simulink model "diplomovka"  (R2014b)
settings: Solver=ode4  StartTime=0.0  StopTime=1000  FixedStep=0.5  RelTol=1e-3
libraries: fuzblock x4
settings Model: Creator=Štefan  LastModifiedBy=Dominik
settings DataIOCC: LimitDataPoints=off

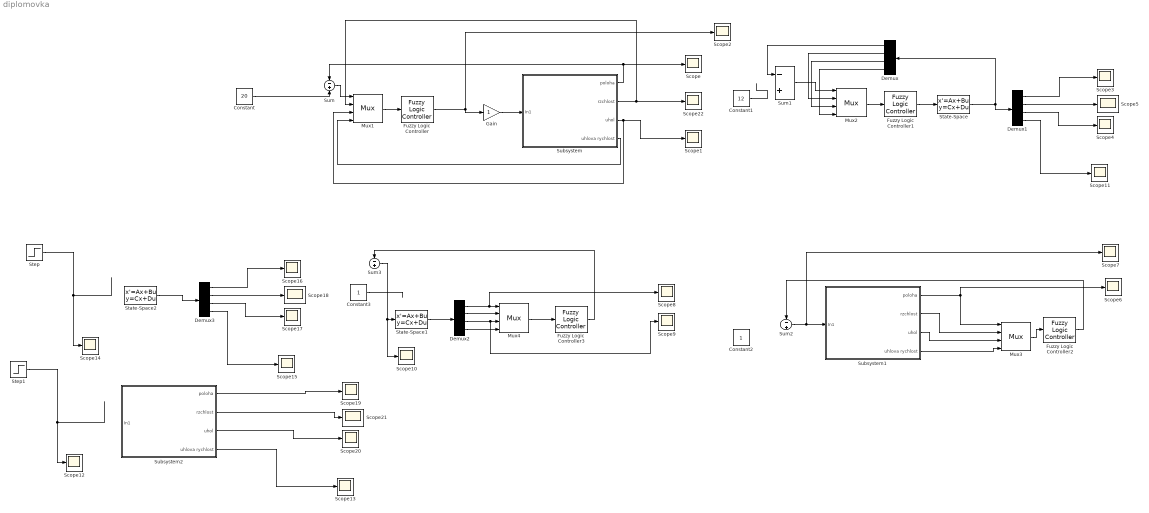
== system diplomovka ==
  Constant : Constant  Value=20
  Constant1 : Constant  Value=12
  Constant2 : Constant
  Constant3 : Constant
  Demux{,1..3} (4 alike) : Demux
  Fuzzy Logic Controller : fuzblock/Fuzzy Logic  Controller  fis=cranemajo
  Fuzzy Logic Controller1 : fuzblock/Fuzzy Logic  Controller  fis=crane
  Fuzzy Logic Controller2 : fuzblock/Fuzzy Logic  Controller  fis=crane
  Fuzzy Logic Controller3 : fuzblock/Fuzzy Logic  Controller  fis=crane
  Gain : Gain
  Mux{1..4} (4 alike) : Mux
  Scope{,1..22} (23 alike) : Scope
      Scope settings: TimeRange=1000  YMin=19.3561872909699  YMax=21.16778149386845
      Scope1 settings: YMin=-0.001  YMax=0.0004
      Scope10 settings: YMin=-0.2  YMax=1  SaveName=ScopeData10
      Scope11 settings: YMin=-0.0004  YMax=0.0004  SaveName=ScopeData11
      Scope12 settings: YMin=-0  YMax=2  SaveName=ScopeData12
      Scope13 settings: YMin=-0.0004  YMax=0.0004  SaveName=ScopeData13
      Scope14 settings: YMin=-0  YMax=2  SaveName=ScopeData14
      Scope15 settings: YMin=-0.0004  YMax=0.0004  SaveName=ScopeData15
      Scope16 settings: SaveName=ScopeData16
      Scope17 settings: SaveName=ScopeData17
      Scope18 settings: SaveName=ScopeData18
      Scope19 settings: SaveName=ScopeData19
      Scope2 settings: YMin=0  YMax=18  SaveName=ScopeData2
      Scope20 settings: SaveName=ScopeData20
      Scope21 settings: SaveName=ScopeData21
      Scope22 settings: TimeRange=150  YMin=0  YMax=25  SaveName=ScopeData22
      Scope3 settings: SaveName=ScopeData3
      Scope4 settings: SaveName=ScopeData4
      Scope5 settings: SaveName=ScopeData5
      Scope6 settings: YMin=-0  YMax=2  SaveName=ScopeData6
      Scope7 settings: YMin=-0  YMax=2  SaveName=ScopeData7
      Scope8 settings: YMin=-0  YMax=2  SaveName=ScopeData8
      Scope9 settings: YMin=-0  YMax=2  SaveName=ScopeData9
  State-Space : StateSpace  A=[0 1 0 0;0 0 Mg/Mk/Z 0;0 0 0 1; 0 0 -(1 + Mg/Mk)/Z 0 ]  B=[0;1;0;-1]./Mk  C=[1 0 0 0;0 1 0 0;0 0 1 0;0 0 0 1]  D=[0;0;0;0]  X0=0
      mask init:
      | Mk=3000;
      | Mg=1500;
      | Z=5/9.81;
  State-Space1 : StateSpace  A=[0 1 0 0;0 0 Mg/Mk/Z 0;0 0 0 1; 0 0 -(1 + Mg/Mk)/Z 0 ]  B=[0;1;0;-1]./Mk  C=[1 0 0 0;0 1 0 0;0 0 1 0;0 0 0 1]  D=[0;0;0;0]  X0=0
      mask init:
      | Mk=3000;
      | Mg=1500;
      | Z=5/9.81;
  State-Space2 : StateSpace  A=[0 1 0 0;0 0 Mg/Mk/Z 0;0 0 0 1; 0 0 -(1 + Mg/Mk)/Z 0 ]  B=[0;1;0;-1]./Mk  C=[1 0 0 0;0 1 0 0;0 0 1 0;0 0 0 1]  D=[0;0;0;0]  X0=0
      mask init:
      | Mk=3000;
      | Mg=1500;
      | Z=5/9.81;
  Step : Step  Time=10  Before=10  After=0  SampleTime=0
  Step1 : Step  Time=10  Before=10  After=0  SampleTime=0
  Subsystem : Subsystem
      mask init:
      | Mk=30;
      | Mg=10;
      | Z=5/9.81;
  Subsystem1 : Subsystem
      mask init:
      | Mk=3000;
      | Mg=1500;
      | Z=5/9.81;
  Subsystem2 : Subsystem
      mask init:
      | Mk=3000;
      | Mg=15000;
      | Z=500/9.81;
  Sum{,1..3} (4 alike) : Sum  Inputs=-+
  wires:
  Subsystem/1("poloha ") -> Scope/1, Sum/1
  Subsystem/2("rzchlost ") -> Mux1/2, Scope22/1
  Subsystem/3("uhol ") -> Mux1/3, Scope1/1
  Fuzzy Logic Controller/1 -> Scope2/1, Gain/1
  Subsystem/4("uhlova rychlost ") -> Mux1/4
  Mux1/1 -> Fuzzy Logic Controller/1
  Sum/1 -> Mux1/1
  State-Space/1 -> Demux/1, Demux1/1
  Fuzzy Logic Controller1/1 -> State-Space/1
  Demux/1 -> Sum1/1
  Mux2/1 -> Fuzzy Logic Controller1/1
  Sum1/1 -> Mux2/1
  Demux/2 -> Mux2/2
  Demux/3 -> Mux2/3
  Demux/4 -> Mux2/4
  Demux1/1 -> Scope3/1
  Demux1/3 -> Scope4/1
  Demux1/2 -> Scope5/1
  Mux3/1 -> Fuzzy Logic Controller2/1
  Subsystem1/1("poloha ") -> Mux3/1, Scope6/1
  Subsystem1/2("rzchlost ") -> Mux3/2
  Subsystem1/3("uhol ") -> Mux3/3
  Subsystem1/4("uhlova rychlost ") -> Mux3/4
  Fuzzy Logic Controller2/1 -> Sum2/1
  Sum2/1 -> Scope7/1, Subsystem1/1(In1)
  Constant3/1 -> ?
  Sum3/1 -> Scope10/1, State-Space1/1
  State-Space1/1 -> Demux2/1
  Demux2/1 -> Scope8/1, Mux4/1
  Demux2/2 -> Mux4/2
  Demux2/3 -> Scope9/1, Mux4/3
  Demux2/4 -> Mux4/4
  Mux4/1 -> Fuzzy Logic Controller3/1
  Fuzzy Logic Controller3/1 -> Sum3/1
  Demux1/4 -> Scope11/1
  Step/1 -> Scope14/1
  Constant/1 -> Sum/2
  State-Space2/1 -> Demux3/1
  Demux3/1 -> Scope16/1
  Demux3/3 -> Scope17/1
  Demux3/2 -> Scope18/1
  Demux3/4 -> Scope15/1
  Step1/1 -> Scope12/1
  Subsystem2/1("poloha ") -> Scope19/1
  Subsystem2/3("uhol ") -> Scope20/1
  Subsystem2/2("rzchlost ") -> Scope21/1
  Subsystem2/4("uhlova rychlost ") -> Scope13/1
  Constant1/1 -> ?
  Gain/1 -> Subsystem/1(In1)

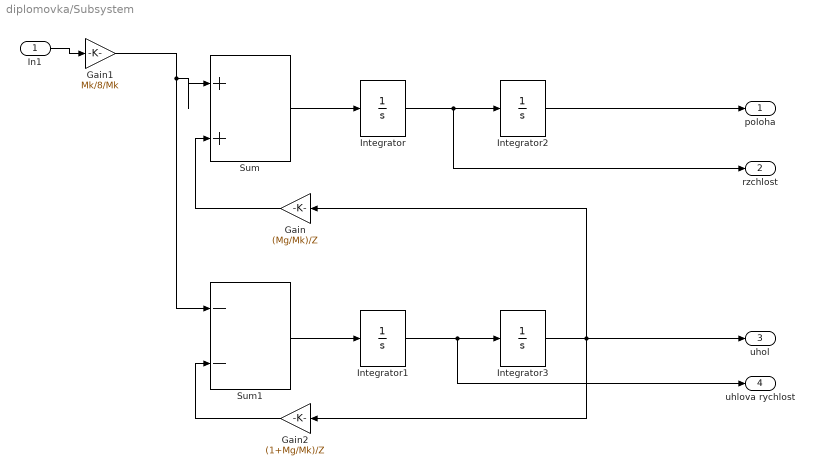
== system diplomovka/Subsystem ==
  In1 : Inport
  Gain : Gain  Gain=(Mg/Mk)/Z
  Gain1 : Gain  Gain=Mk/8/Mk
  Gain2 : Gain  Gain=(1+Mg/Mk)/Z
  Integrator{,1..3} (4 alike) : Integrator
  Sum : Sum  Inputs=|++
  Sum1 : Sum  Inputs=--
  "poloha " : Outport
  "rzchlost " : Outport  Port=2
  "uhol " : Outport  Port=3
  "uhlova rychlost " : Outport  Port=4
  wires:
  Sum1/1 -> Integrator1/1
  Sum/1 -> Integrator/1
  Integrator2/1 -> "poloha "/1
  Integrator3/1 -> "uhol "/1, Gain2/1, Gain/1
  Integrator1/1 -> "uhlova rychlost "/1, Integrator3/1
  Gain2/1 -> Sum1/2
  Gain/1 -> Sum/2
  In1/1 -> Gain1/1
  Integrator/1 -> "rzchlost "/1, Integrator2/1
  Gain1/1 -> Sum1/1, Sum/1

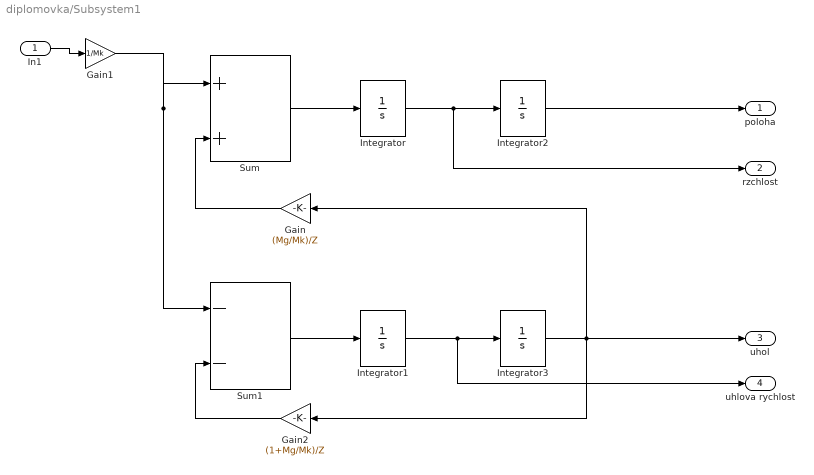
== system diplomovka/Subsystem1 ==
  In1 : Inport
  Gain : Gain  Gain=(Mg/Mk)/Z
  Gain1 : Gain  Gain=1/Mk
  Gain2 : Gain  Gain=(1+Mg/Mk)/Z
  Integrator{,1..3} (4 alike) : Integrator
  Sum : Sum  Inputs=|++
  Sum1 : Sum  Inputs=--
  "poloha " : Outport
  "rzchlost " : Outport  Port=2
  "uhol " : Outport  Port=3
  "uhlova rychlost " : Outport  Port=4
  wires:
  Integrator/1 -> Integrator2/1, "rzchlost "/1
  In1/1 -> Gain1/1
  Gain/1 -> Sum/2
  Gain2/1 -> Sum1/2
  Gain1/1 -> Sum/1, Sum1/1
  Integrator1/1 -> Integrator3/1, "uhlova rychlost "/1
  Integrator3/1 -> Gain/1, Gain2/1, "uhol "/1
  Integrator2/1 -> "poloha "/1
  Sum/1 -> Integrator/1
  Sum1/1 -> Integrator1/1

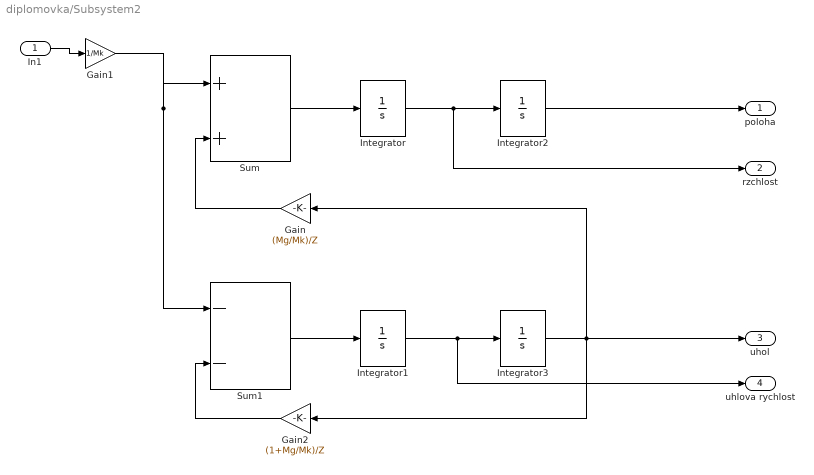
== system diplomovka/Subsystem2 ==
  In1 : Inport
  Gain : Gain  Gain=(Mg/Mk)/Z
  Gain1 : Gain  Gain=1/Mk
  Gain2 : Gain  Gain=(1+Mg/Mk)/Z
  Integrator{,1..3} (4 alike) : Integrator
  Sum : Sum  Inputs=|++
  Sum1 : Sum  Inputs=--
  "poloha " : Outport
  "rzchlost " : Outport  Port=2
  "uhol " : Outport  Port=3
  "uhlova rychlost " : Outport  Port=4
  wires:
  Integrator/1 -> Integrator2/1, "rzchlost "/1
  In1/1 -> Gain1/1
  Gain/1 -> Sum/2
  Gain2/1 -> Sum1/2
  Gain1/1 -> Sum/1, Sum1/1
  Integrator1/1 -> Integrator3/1, "uhlova rychlost "/1
  Integrator3/1 -> Gain/1, Gain2/1, "uhol "/1
  Integrator2/1 -> "poloha "/1
  Sum/1 -> Integrator/1
  Sum1/1 -> Integrator1/1
